simulink model "Masse_MultirotorSimHinf"  (R2018b)
settings: Solver=VariableStepAuto  StartTime=0.0  StopTime=Simulation.T_END  MaxStep=Simulation.TS_MAX  RelTol=1e-3  EnableMultiTasking=on
PreLoadFcn:
  | % InitializeParameters;
undefined symbols (not defined in the file): Aero, armed, ctrl_state, INIT_PARAM_VECTOR, Initial, K_i, K_p, Motor, mpc_att_sp, mpc_ctrl_state, mpc_manual, mpc_pos_sp_triplet, mpc_vehicle_land_detected, mpc_vehicle_status, Simulation, SOF1, SOF2, Uav, Upsilon, v_att_sp, v_control_mode
libraries: simulink_extras x9, simulink x6, dspstat3 x1, Px4Library x1
(part 9 of 11)

== matlab function Masse_MultirotorSimHinf/Sensor Model/Global reprojection/map_projection_reproject ==
  data: x input; y input; lat output; lon output; LAT0 parameter; LON0 parameter
function [ lat, lon ] = map_projection_reproject( x, y, LAT0, LON0)
%#codegen
%MAP_PROJECTION_REPROJECT
    M_DEG_TO_RAD = 0.017453292519943295;
	ref.lat_rad = LAT0 * M_DEG_TO_RAD;
	ref.lon_rad = LON0 * M_DEG_TO_RAD;
	ref.sin_lat = 0;
	ref.cos_lat = 0; 
    ref.sin_lat = sin(ref.lat_rad);
    ref.cos_lat = cos(ref.lat_rad);
    
    CONSTANTS_RADIUS_OF_EARTH = 6371000;
    M_PI = 3.14159265358979323846;

    x_rad = x / CONSTANTS_RADIUS_OF_EARTH;
    y_rad = y / CONSTANTS_RADIUS_OF_EARTH;
    c = sqrt(x_rad * x_rad + y_rad * y_rad);
    
    sin_c = sin(c);
    cos_c = cos(c);

    if (abs(c) > eps)
        lat_rad = asin(cos_c * ref.sin_lat + (x_rad * sin_c * ref.cos_lat) / c);
        lon_rad = (ref.lon_rad + atan2(y_rad * sin_c, c * ref.cos_lat * cos_c - x_rad * ref.sin_lat * sin_c));
    else
        lat_rad = ref.lat_rad;
        lon_rad = ref.lon_rad;
    end

    lat = lat_rad * 180.0 / M_PI;
    lon = lon_rad * 180.0 / M_PI;
end

== matlab function Masse_MultirotorSimHinf/Quadrotor Quaternion Model/Compute S Matrix2/MATLAB Function ==
  data: q input; S output
function S = ComputeSMatrix(q)
%COMPUTESMATRIX Compute S Matrix
%   Written by:    J.X.J. Bannwarth, 2017/03/28
%   Last modified: J.X.J. Bannwarth, 2018/12/11
    S = zeros( 4, 3 );
    S(1,1) = -q(2) * 0.5;
    S(1,2) = -q(3) * 0.5;
    S(1,3) = -q(4) * 0.5;
    S(2,1) =  q(1) * 0.5;
    S(2,2) = -q(4) * 0.5;
    S(2,3) =  q(3) * 0.5;
    S(3,1) =  q(4) * 0.5;
    S(3,2) =  q(1) * 0.5;
    S(3,3) = -q(2) * 0.5;
    S(4,1) = -q(3) * 0.5;
    S(4,2) =  q(2) * 0.5;
    S(4,3) =  q(1) * 0.5;
end

== matlab function Masse_MultirotorSimHinf/Sensor Model/Quaternion to Euler Angles/MATLAB Function ==
  data: quat input; eul output
function eul   = QuaternionToEuler( quat )
%QUATERNIONTOEULER Convert quaternion to euler angles
%   Based on PX4 Firmware code: https://github.com/PX4/Firmware
%   Written by:    J.X.J. Bannwarth, 2016/08/29
%   Last modified: J.X.J. Bannwarth, 2018/12/11

    eul = [ atan2(2.0 .* (quat(1) .* quat(2) + quat(3) .* quat(4)), ...
                1.0 - 2.0 .* (quat(2) .* quat(2) + quat(3) .* quat(3)));
	        asin(2.0 .* (quat(1) .* quat(3) - quat(4) .* quat(2)));
            atan2(2.0 .* (quat(1) .* quat(4) + quat(2) .* quat(3)), ...
                1.0 - 2.0 .* (quat(3) .* quat(3) + quat(4) .* quat(4))) ];
end

== matlab function Masse_MultirotorSimHinf/Quadrotor Quaternion Model/Compute S Matrix1/MATLAB Function ==
  data: q input; S output
function S = ComputeSMatrix(q)
%COMPUTESMATRIX Compute S Matrix
%   Written by:    J.X.J. Bannwarth, 2017/03/28
%   Last modified: J.X.J. Bannwarth, 2018/12/11
    S = zeros( 4, 3 );
    S(1,1) = -q(2) * 0.5;
    S(1,2) = -q(3) * 0.5;
    S(1,3) = -q(4) * 0.5;
    S(2,1) =  q(1) * 0.5;
    S(2,2) = -q(4) * 0.5;
    S(2,3) =  q(3) * 0.5;
    S(3,1) =  q(4) * 0.5;
    S(3,2) =  q(1) * 0.5;
    S(3,3) = -q(2) * 0.5;
    S(4,1) = -q(3) * 0.5;
    S(4,2) =  q(2) * 0.5;
    S(4,3) =  q(1) * 0.5;
end

== matlab function Masse_MultirotorSimHinf/Sensor Model/attitude_estimator_q/Input assignment q ==
  data: airspeed_sub_indicated_airspeed_m_s input; airspeed_sub_timestamp input; global_pos_sub_eph input; global_pos_sub_lat input; global_pos_sub_lon input; global_pos_sub_timestamp input; global_pos_sub_vel_n input; global_pos_sub_vel_e input; global_pos_sub_vel_d input; mocap_sub_q input; mocap_sub_timestamp input; sensors_sub_timestamp input; sensors_sub_gyro_rad input; sensors_sub_accelerometer_m_s2 input; sensors_sub_accelerometer_timestamp_relative input; sensors_sub_magnetometer_ga input; sensors_sub_magnetometer_timestamp_relative input; selfVecIn input; selfVec output
function selfVec = InputAssignment( ...
	     airspeed_sub_indicated_airspeed_m_s, ...
	                  airspeed_sub_timestamp, ...
	                      global_pos_sub_eph, ...
	                      global_pos_sub_lat, ...
	                      global_pos_sub_lon, ...
	                global_pos_sub_timestamp, ...
	                    global_pos_sub_vel_n, ...
	                    global_pos_sub_vel_e, ...
	                    global_pos_sub_vel_d, ...
	                             mocap_sub_q, ...
	                     mocap_sub_timestamp, ...
	                   sensors_sub_timestamp, ...
	                    sensors_sub_gyro_rad, ...
	          sensors_sub_accelerometer_m_s2, ...
	sensors_sub_accelerometer_timestamp_relative, ...
	             sensors_sub_magnetometer_ga, ...
	sensors_sub_magnetometer_timestamp_relative, ...
	                               selfVecIn ...
	)
%#codegen

	selfVec = selfVecIn;

	% Variable assignment
	selfVec(10:10) =      airspeed_sub_indicated_airspeed_m_s;
	selfVec(11:11) =                   airspeed_sub_timestamp;
	selfVec(45:45) =                       global_pos_sub_eph;
	selfVec(46:46) =                       global_pos_sub_lat;
	selfVec(47:47) =                       global_pos_sub_lon;
	selfVec(48:48) =                 global_pos_sub_timestamp;
	selfVec(50:50) =                     global_pos_sub_vel_n;
	selfVec(51:51) =                     global_pos_sub_vel_e;
	selfVec(52:52) =                     global_pos_sub_vel_d;
	selfVec(147:150) =                              mocap_sub_q;
	selfVec(151:151) =                      mocap_sub_timestamp;
	selfVec(166:166) =                    sensors_sub_timestamp;
	selfVec(168:170) =                     sensors_sub_gyro_rad;
	selfVec(171:173) =           sensors_sub_accelerometer_m_s2;
	selfVec(174:174) = sensors_sub_accelerometer_timestamp_relative;
	selfVec(175:177) =              sensors_sub_magnetometer_ga;
	selfVec(178:178) = sensors_sub_magnetometer_timestamp_relative;
end

== matlab function Masse_MultirotorSimHinf/Sensor Model/attitude_estimator_q/Output selection q ==
  data: att_pub_timestamp output; att_pub_rollspeed output; att_pub_pitchspeed output; att_pub_yawspeed output; att_pub_q output; selfVec input; ctrl_state_pub_x_acc output; ctrl_state_pub_y_acc output; ctrl_state_pub_z_acc output
function [ ...
                        att_pub_timestamp, ...
                        att_pub_rollspeed, ...
                       att_pub_pitchspeed, ...
                         att_pub_yawspeed, ...
                                att_pub_q, ...
                     ctrl_state_pub_x_acc, ...
                     ctrl_state_pub_y_acc, ...
                     ctrl_state_pub_z_acc] ...
   = OutputSelection( selfVec )
%#codegen

	% Variable assignment
	                       att_pub_timestamp = selfVec(14:14);
	                       att_pub_rollspeed = selfVec(15:15);
	                      att_pub_pitchspeed = selfVec(16:16);
	                        att_pub_yawspeed = selfVec(17:17);
	                               att_pub_q = selfVec(18:21);
	                    ctrl_state_pub_x_acc = selfVec(29:29);
	                    ctrl_state_pub_y_acc = selfVec(30:30);
	                    ctrl_state_pub_z_acc = selfVec(31:31);
end
